simulink model "TCDT"  (R2019b)
settings: Solver=FixedStepAuto  StartTime=0.0  StopTime=tstop  FixedStep=tstep  RelTol=1e-3
values from neighbouring files (symbols this model uses):
  tstep = 0.01    [data.m]
  xic = [0 0]    [data.m]
settings Model: Creator=WIN10  LastModifiedBy=Ram Padmanabhan
settings DataIOCC: SaveOutput=off  SignalLogging=off  DSMLogging=off  SaveTime=off  ReturnWorkspaceOutputs=off

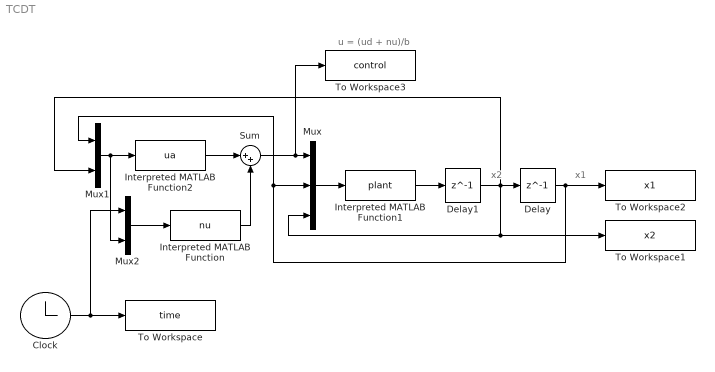
== system TCDT ==
  note: u = (ud + nu)/b
  note: x2
  note: x1
  Clock : Clock
  Delay : Delay  DelayLength=1  InitialCondition=xic(1)  SampleTime=tstep
  Delay1 : Delay  DelayLength=1  InitialCondition=xic(2)  SampleTime=tstep
  Interpreted MATLAB Function : MATLABFcn  MATLABFcn=nu  OutputDimensions=1
  Interpreted MATLAB Function1 : MATLABFcn  MATLABFcn=plant  OutputDimensions=1
  Interpreted MATLAB Function2 : MATLABFcn  MATLABFcn=ua  OutputDimensions=1
  Mux : Mux  Inputs=3
  Mux1 : Mux  Inputs=2
  Mux2 : Mux  Inputs=2
  Sum : Sum  Inputs=|++
  To Workspace : ToWorkspace  VariableName=time  SampleTime=-1
  To Workspace1 : ToWorkspace  VariableName=x2  SampleTime=-1
  To Workspace2 : ToWorkspace  VariableName=x1  SampleTime=-1
  To Workspace3 : ToWorkspace  VariableName=control  SampleTime=-1
  wires:
  Clock/1 -> Mux2/1, To Workspace/1
  Delay1/1 -> Mux/3, To Workspace1/1, Mux1/2, Delay/1
  Delay/1 -> Mux1/1, Mux/2, To Workspace2/1
  Interpreted MATLAB Function1/1 -> Delay1/1
  Mux/1 -> Interpreted MATLAB Function1/1
  Sum/1 -> To Workspace3/1, Mux/1
  Interpreted MATLAB Function2/1 -> Sum/1
  Interpreted MATLAB Function/1 -> Sum/2
  Mux1/1 -> Mux2/2, Interpreted MATLAB Function2/1
  Mux2/1 -> Interpreted MATLAB Function/1
